simulink model "sampleModel7288_pp_1_1"  (R2018a)
settings: Solver=VariableStepAuto  StartTime=0.0  StopTime=10.0  RelTol=1e-3
undefined symbols (not defined in the file): DiscIntNeverNeededParam, sigbuilder_block
libraries: simulink x497
(part 4 of 10)

== system sampleModel7288_pp_1_1/cfblk286 ==
  cfblk1 : Inport
  Action Port : ActionPort  ActionType=then
  cfblk{10..13} (4 alike) : Delay
  cfblk3 : simulink/Continuous/PID Controller (2DOF)  Controller=PID  TimeDomain=Discrete-time  SampleTime=-1  IntegratorMethod=Forward Euler  FilterMethod=Forward Euler  Form=Parallel  UseFilter=on  ControllerParametersSource=internal  P=1  I=1  D=0  N=100  b=1  c=1  InitialConditionSource=internal  InitialConditionForIntegrator=0  InitialConditionForFilter=0  ExternalReset=none  LimitOutput=off  UpperSaturationLimit=inf  LowerSaturationLimit=-inf  LinearizeAsGain=off  AntiWindupMode=none  Kb=1  TrackingMode=off  Kt=1  PParamMin=[]  PParamMax=[]  IParamMin=[]  IParamMax=[]  DParamMin=[]  DParamMax=[]  NParamMin=[]  NParamMax=[]  bParamMin=[]  bParamMax=[]  cParamMin=[]  cParamMax=[]  KbParamMin=[]  KbParamMax=[]  KtParamMin=[]  KtParamMax=[]  POutMin=[]  POutMax=[]  IOutMin=[]  IOutMax=[]  DOutMin=[]  DOutMax=[]  NOutMin=[]  NOutMax=[]  bOutMin=[]  bOutMax=[]  cOutMin=[]  cOutMax=[]  KbOutMin=[]  KbOutMax=[]  KtOutMin=[]  KtOutMax=[]  IntegratorOutMin=[]  IntegratorOutMax=[]  FilterOutMin=[]  FilterOutMax=[]  SumOutMin=[]  SumOutMax=[]  Sum1OutMin=[]  Sum1OutMax=[]  Sum2OutMin=[]  Sum2OutMax=[]  Sum3OutMin=[]  Sum3OutMax=[]  SumI1OutMin=[]  SumI1OutMax=[]  SumI2OutMin=[]  SumI2OutMax=[]  SumI3OutMin=[]  SumI3OutMax=[]  SumDOutMin=[]  SumDOutMax=[]  SaturationOutMin=[]  SaturationOutMax=[]  IntegratorContinuousStateAttributes=''  IntegratorStateMustResolveToSignalObject=off  IntegratorRTWStateStorageClass=Auto  FilterContinuousStateAttributes=''  FilterStateMustResolveToSignalObject=off  FilterRTWStateStorageClass=Auto  DifferentiatorICPrevScaledInput=0  DifferentiatorOutMin=[]  DifferentiatorOutMax=[]  FilterDiffOutCoefMin=[]  FilterDiffOutCoefMax=[]  SumDenOutMin=[]  SumDenOutMax=[]  SumNumOutMin=[]  SumNumOutMax=[]  ReciprocalOutMin=[]  ReciprocalOutMax=[]  DivideOutMin=[]  DivideOutMax=[]  TunerSelectOption=Transfer Function Based (PID Tuner App)
  cfblk4 : DiscreteFilter
  cfblk5 : DiscreteZeroPole  Poles=[0 0.5]  Gain=1  SampleTime=-1
  cfblk6 : Delay  DelayLengthSource=Input port
      settings: InputPortMap=u0,p1
  cfblk7 : simulink/Continuous/PID Controller (2DOF)  Controller=PID  TimeDomain=Discrete-time  SampleTime=-1  IntegratorMethod=Forward Euler  FilterMethod=Forward Euler  Form=Parallel  UseFilter=on  ControllerParametersSource=internal  P=1  I=1  D=0  N=100  b=1  c=1  InitialConditionSource=internal  InitialConditionForIntegrator=0  InitialConditionForFilter=0  ExternalReset=none  LimitOutput=off  UpperSaturationLimit=inf  LowerSaturationLimit=-inf  LinearizeAsGain=off  AntiWindupMode=none  Kb=1  TrackingMode=off  Kt=1  PParamMin=[]  PParamMax=[]  IParamMin=[]  IParamMax=[]  DParamMin=[]  DParamMax=[]  NParamMin=[]  NParamMax=[]  bParamMin=[]  bParamMax=[]  cParamMin=[]  cParamMax=[]  KbParamMin=[]  KbParamMax=[]  KtParamMin=[]  KtParamMax=[]  POutMin=[]  POutMax=[]  IOutMin=[]  IOutMax=[]  DOutMin=[]  DOutMax=[]  NOutMin=[]  NOutMax=[]  bOutMin=[]  bOutMax=[]  cOutMin=[]  cOutMax=[]  KbOutMin=[]  KbOutMax=[]  KtOutMin=[]  KtOutMax=[]  IntegratorOutMin=[]  IntegratorOutMax=[]  FilterOutMin=[]  FilterOutMax=[]  SumOutMin=[]  SumOutMax=[]  Sum1OutMin=[]  Sum1OutMax=[]  Sum2OutMin=[]  Sum2OutMax=[]  Sum3OutMin=[]  Sum3OutMax=[]  SumI1OutMin=[]  SumI1OutMax=[]  SumI2OutMin=[]  SumI2OutMax=[]  SumI3OutMin=[]  SumI3OutMax=[]  SumDOutMin=[]  SumDOutMax=[]  SaturationOutMin=[]  SaturationOutMax=[]  IntegratorContinuousStateAttributes=''  IntegratorStateMustResolveToSignalObject=off  IntegratorRTWStateStorageClass=Auto  FilterContinuousStateAttributes=''  FilterStateMustResolveToSignalObject=off  FilterRTWStateStorageClass=Auto  DifferentiatorICPrevScaledInput=0  DifferentiatorOutMin=[]  DifferentiatorOutMax=[]  FilterDiffOutCoefMin=[]  FilterDiffOutCoefMax=[]  SumDenOutMin=[]  SumDenOutMax=[]  SumNumOutMin=[]  SumNumOutMax=[]  ReciprocalOutMin=[]  ReciprocalOutMax=[]  DivideOutMin=[]  DivideOutMax=[]  TunerSelectOption=Transfer Function Based (PID Tuner App)
  cyemi_{778..789} (12 alike) : DataTypeConversion  OutDataTypeStr=double
  cfblk2 : Outport
  cfblk8 : Outport  Port=2
  cfblk9 : Outport  Port=3
  wires:
  cfblk5/1 -> cfblk2/1, cyemi_778/1, cyemi_779/1, cyemi_784/1
  cfblk1/1 -> cfblk9/1
  cfblk6/1 -> cfblk8/1, cyemi_781/1, cyemi_785/1
  cyemi_778/1 -> cfblk10/1
  cyemi_779/1 -> cfblk11/1
  cyemi_780/1 -> cfblk12/1
  cfblk4/1 -> cyemi_780/1
  cyemi_781/1 -> cfblk13/1
  cyemi_782/1 -> cfblk3/1
  cfblk10/1 -> cyemi_782/1
  cyemi_783/1 -> cfblk3/2
  cfblk13/1 -> cyemi_783/1
  cyemi_784/1 -> cfblk4/1
  cyemi_785/1 -> cfblk5/1
  cyemi_786/1 -> cfblk6/1
  cfblk12/1 -> cyemi_786/1
  cyemi_787/1 -> cfblk6/2
  cfblk7/1 -> cyemi_787/1
  cyemi_788/1 -> cfblk7/1
  cfblk3/1 -> cyemi_788/1
  cyemi_789/1 -> cfblk7/2
  cfblk11/1 -> cyemi_789/1

== system sampleModel7288_pp_1_1/cfblk287 ==
  cfblk1 : Inport
  cfblk11 : Inport  Port=2
  cfblk12 : Inport  Port=3
  Action Port : ActionPort  ActionType=else
  cfblk10 : simulink/Continuous/PID Controller  Controller=PID  TimeDomain=Discrete-time  SampleTime=-1  IntegratorMethod=Forward Euler  FilterMethod=Forward Euler  Form=Parallel  UseFilter=on  ControllerParametersSource=internal  P=1  I=1  D=0  N=100  InitialConditionSource=internal  InitialConditionForIntegrator=0  InitialConditionForFilter=0  ExternalReset=none  LimitOutput=off  UpperSaturationLimit=inf  LowerSaturationLimit=-inf  LinearizeAsGain=off  AntiWindupMode=none  Kb=1  TrackingMode=off  Kt=1  PParamMin=[]  PParamMax=[]  IParamMin=[]  IParamMax=[]  DParamMin=[]  DParamMax=[]  NParamMin=[]  NParamMax=[]  KbParamMin=[]  KbParamMax=[]  KtParamMin=[]  KtParamMax=[]  POutMin=[]  POutMax=[]  IOutMin=[]  IOutMax=[]  DOutMin=[]  DOutMax=[]  NOutMin=[]  NOutMax=[]  KbOutMin=[]  KbOutMax=[]  KtOutMin=[]  KtOutMax=[]  IntegratorOutMin=[]  IntegratorOutMax=[]  FilterOutMin=[]  FilterOutMax=[]  SumOutMin=[]  SumOutMax=[]  SumI1OutMin=[]  SumI1OutMax=[]  SumI2OutMin=[]  SumI2OutMax=[]  SumI3OutMin=[]  SumI3OutMax=[]  SumDOutMin=[]  SumDOutMax=[]  SaturationOutMin=[]  SaturationOutMax=[]  IntegratorContinuousStateAttributes=''  IntegratorStateMustResolveToSignalObject=off  IntegratorRTWStateStorageClass=Auto  FilterContinuousStateAttributes=''  FilterStateMustResolveToSignalObject=off  FilterRTWStateStorageClass=Auto  DifferentiatorICPrevScaledInput=0  DifferentiatorOutMin=[]  DifferentiatorOutMax=[]  FilterDiffOutCoefMin=[]  FilterDiffOutCoefMax=[]  SumDenOutMin=[]  SumDenOutMax=[]  SumNumOutMin=[]  SumNumOutMax=[]  ReciprocalOutMin=[]  ReciprocalOutMax=[]  DivideOutMin=[]  DivideOutMax=[]  TunerSelectOption=Transfer Function Based (PID Tuner App)
  cfblk15 : Delay
  cfblk16 : Delay
  cfblk3 : DiscreteTransferFcn
  cfblk4 : DiscreteIntegrator  SampleTime=-1  OutDataTypeStr=double  ICPrevOutput=DiscIntNeverNeededParam  ICPrevScaledInput=DiscIntNeverNeededParam
  cfblk5 : Delay  DelayLengthSource=Input port
      settings: InputPortMap=u0,p1
  cfblk6 : Delay  DelayLengthSource=Input port
      settings: InputPortMap=u0,p1
  cfblk7 : simulink/Discrete/Tapped Delay  vinit=0.0  samptime=-1  NumDelays=1  DelayOrder=Oldest  includeCurrent=off
  cfblk8 : simulink/Discrete/Difference  ICPrevInput=0.0  OutMin=[]  OutMax=[]  OutDataTypeStr=double  OutputDataTypeScalingMode=double  OutDataType=fixdt(1, 16)  OutScaling=2^-10  DoSatur=off
  cfblk9 : DiscreteStateSpace  SampleTime=-1
  cyemi_{793..804} (12 alike) : DataTypeConversion  OutDataTypeStr=double
  cfblk2 : Outport
  cfblk13 : Outport  Port=2
  cfblk14 : Outport  Port=3
  wires:
  cfblk7/1 -> cfblk13/1
  cfblk11/1 -> cyemi_798/1, cyemi_802/1
  cfblk1/1 -> cfblk2/1
  cfblk9/1 -> cfblk14/1
  cfblk8/1 -> cyemi_795/1, cyemi_797/1
  cyemi_793/1 -> cfblk10/1
  cfblk5/1 -> cyemi_793/1
  cyemi_794/1 -> cfblk15/1
  cfblk6/1 -> cyemi_794/1
  cyemi_795/1 -> cfblk16/1
  cyemi_796/1 -> cfblk3/1
  cfblk15/1 -> cyemi_796/1
  cyemi_797/1 -> cfblk4/1
  cyemi_798/1 -> cfblk5/1
  cyemi_799/1 -> cfblk5/2
  cfblk16/1 -> cyemi_799/1
  cyemi_800/1 -> cfblk6/1
  cfblk3/1 -> cyemi_800/1
  cyemi_801/1 -> cfblk6/2
  cfblk12/1 -> cyemi_801/1
  cyemi_802/1 -> cfblk7/1
  cyemi_803/1 -> cfblk8/1
  cfblk10/1 -> cyemi_803/1
  cyemi_804/1 -> cfblk9/1
  cfblk4/1 -> cyemi_804/1

== system sampleModel7288_pp_1_1/cfblk288 ==
  cfblk1 : Inport
  cfblk11 : Inport  Port=2
  Action Port : ActionPort  ActionType=then
  cfblk10 : If  SampleTime=1
  cfblk15 : Subsystem  TreatAsAtomicUnit=on
  cfblk16 : Subsystem  TreatAsAtomicUnit=on
  cfblk17 : Delay
  cfblk18 : Delay
  cfblk19 : Delay
  cfblk3 : simulink/Continuous/PID Controller  Controller=PID  TimeDomain=Discrete-time  SampleTime=-1  IntegratorMethod=Forward Euler  FilterMethod=Forward Euler  Form=Parallel  UseFilter=on  ControllerParametersSource=internal  P=1  I=1  D=0  N=100  InitialConditionSource=internal  InitialConditionForIntegrator=0  InitialConditionForFilter=0  ExternalReset=none  LimitOutput=off  UpperSaturationLimit=inf  LowerSaturationLimit=-inf  LinearizeAsGain=off  AntiWindupMode=none  Kb=1  TrackingMode=off  Kt=1  PParamMin=[]  PParamMax=[]  IParamMin=[]  IParamMax=[]  DParamMin=[]  DParamMax=[]  NParamMin=[]  NParamMax=[]  KbParamMin=[]  KbParamMax=[]  KtParamMin=[]  KtParamMax=[]  POutMin=[]  POutMax=[]  IOutMin=[]  IOutMax=[]  DOutMin=[]  DOutMax=[]  NOutMin=[]  NOutMax=[]  KbOutMin=[]  KbOutMax=[]  KtOutMin=[]  KtOutMax=[]  IntegratorOutMin=[]  IntegratorOutMax=[]  FilterOutMin=[]  FilterOutMax=[]  SumOutMin=[]  SumOutMax=[]  SumI1OutMin=[]  SumI1OutMax=[]  SumI2OutMin=[]  SumI2OutMax=[]  SumI3OutMin=[]  SumI3OutMax=[]  SumDOutMin=[]  SumDOutMax=[]  SaturationOutMin=[]  SaturationOutMax=[]  IntegratorContinuousStateAttributes=''  IntegratorStateMustResolveToSignalObject=off  IntegratorRTWStateStorageClass=Auto  FilterContinuousStateAttributes=''  FilterStateMustResolveToSignalObject=off  FilterRTWStateStorageClass=Auto  DifferentiatorICPrevScaledInput=0  DifferentiatorOutMin=[]  DifferentiatorOutMax=[]  FilterDiffOutCoefMin=[]  FilterDiffOutCoefMax=[]  SumDenOutMin=[]  SumDenOutMax=[]  SumNumOutMin=[]  SumNumOutMax=[]  ReciprocalOutMin=[]  ReciprocalOutMax=[]  DivideOutMin=[]  DivideOutMax=[]  TunerSelectOption=Transfer Function Based (PID Tuner App)
  cfblk4 : DiscreteStateSpace  SampleTime=-1
  cfblk5 : simulink/Discrete/Tapped Delay  vinit=0.0  samptime=-1  NumDelays=1  DelayOrder=Oldest  includeCurrent=off
  cfblk6 : Delay  DelayLengthSource=Input port
      settings: InputPortMap=u0,p1
  cfblk7 : Delay  DelayLengthSource=Input port
      settings: InputPortMap=u0,p1
  cfblk8 : UnitDelay  SampleTime=-1
  cfblk9 : UnitDelay  SampleTime=-1
  cyemi_{807..808,820..821,828..834,836..839} (15 alike) : DataTypeConversion  OutDataTypeStr=double
  cyemi_835 : DataTypeConversion  OutDataTypeStr=uint32
  cfblk2 : Outport
  cfblk12 : Outport  Port=2
  cfblk13 : Outport  Port=3
  cfblk14 : Outport  Port=4
  wires:
  cfblk15/1(cfblk2) -> cfblk2/1
  cfblk6/1 -> cyemi_828/1, cyemi_839/1
  cfblk9/1 -> cfblk12/1, cyemi_838/1
  cfblk8/1 -> cfblk13/1
  cfblk15/2(cfblk11) -> cyemi_829/1, cyemi_837/1
  cfblk3/1 -> cfblk14/1, cyemi_821/1, cyemi_836/1
  cfblk10/1 -> cfblk15/Action
  cfblk10/2 -> cfblk16/Action
  cyemi_807/1 -> cfblk10/1
  cfblk19/1 -> cyemi_807/1
  cyemi_808/1 -> cfblk15/1(cfblk1)
  cfblk17/1 -> cyemi_808/1
  cyemi_820/1 -> cfblk16/1(cfblk1)
  cfblk18/1 -> cyemi_820/1
  cyemi_821/1 -> cfblk16/2(cfblk8)
  cyemi_828/1 -> cfblk17/1
  cyemi_829/1 -> cfblk18/1
  cyemi_830/1 -> cfblk19/1
  cfblk4/1 -> cyemi_830/1
  cyemi_831/1 -> cfblk3/1
  cfblk5/1 -> cyemi_831/1
  cyemi_832/1 -> cfblk4/1
  cfblk7/1 -> cyemi_832/1
  cyemi_833/1 -> cfblk5/1
  cfblk1/1 -> cyemi_833/1
  cyemi_834/1 -> cfblk6/1
  cfblk16/1(cfblk2) -> cyemi_834/1
  cyemi_835/1 -> cfblk6/2
  cfblk11/1 -> cyemi_835/1
  cyemi_836/1 -> cfblk7/1
  cyemi_837/1 -> cfblk7/2
  cyemi_838/1 -> cfblk8/1
  cyemi_839/1 -> cfblk9/1

== system sampleModel7288_pp_1_1/cfblk289 ==
  cfblk1 : Inport
  Action Port : ActionPort  ActionType=else
  cfblk3 : simulink/Continuous/PID Controller  Controller=PID  TimeDomain=Discrete-time  SampleTime=-1  IntegratorMethod=Forward Euler  FilterMethod=Forward Euler  Form=Parallel  UseFilter=on  ControllerParametersSource=internal  P=1  I=1  D=0  N=100  InitialConditionSource=internal  InitialConditionForIntegrator=0  InitialConditionForFilter=0  ExternalReset=none  LimitOutput=off  UpperSaturationLimit=inf  LowerSaturationLimit=-inf  LinearizeAsGain=off  AntiWindupMode=none  Kb=1  TrackingMode=off  Kt=1  PParamMin=[]  PParamMax=[]  IParamMin=[]  IParamMax=[]  DParamMin=[]  DParamMax=[]  NParamMin=[]  NParamMax=[]  KbParamMin=[]  KbParamMax=[]  KtParamMin=[]  KtParamMax=[]  POutMin=[]  POutMax=[]  IOutMin=[]  IOutMax=[]  DOutMin=[]  DOutMax=[]  NOutMin=[]  NOutMax=[]  KbOutMin=[]  KbOutMax=[]  KtOutMin=[]  KtOutMax=[]  IntegratorOutMin=[]  IntegratorOutMax=[]  FilterOutMin=[]  FilterOutMax=[]  SumOutMin=[]  SumOutMax=[]  SumI1OutMin=[]  SumI1OutMax=[]  SumI2OutMin=[]  SumI2OutMax=[]  SumI3OutMin=[]  SumI3OutMax=[]  SumDOutMin=[]  SumDOutMax=[]  SaturationOutMin=[]  SaturationOutMax=[]  IntegratorContinuousStateAttributes=''  IntegratorStateMustResolveToSignalObject=off  IntegratorRTWStateStorageClass=Auto  FilterContinuousStateAttributes=''  FilterStateMustResolveToSignalObject=off  FilterRTWStateStorageClass=Auto  DifferentiatorICPrevScaledInput=0  DifferentiatorOutMin=[]  DifferentiatorOutMax=[]  FilterDiffOutCoefMin=[]  FilterDiffOutCoefMax=[]  SumDenOutMin=[]  SumDenOutMax=[]  SumNumOutMin=[]  SumNumOutMax=[]  ReciprocalOutMin=[]  ReciprocalOutMax=[]  DivideOutMin=[]  DivideOutMax=[]  TunerSelectOption=Transfer Function Based (PID Tuner App)
  cfblk4 : DiscreteStateSpace  SampleTime=-1
  cfblk5 : DiscreteStateSpace  SampleTime=-1
  cfblk6 : simulink/Discrete/Tapped Delay  vinit=0.0  samptime=-1  NumDelays=1  DelayOrder=Oldest  includeCurrent=off
  cfblk7 : DiscreteIntegrator  SampleTime=-1  OutDataTypeStr=double  ICPrevOutput=DiscIntNeverNeededParam  ICPrevScaledInput=DiscIntNeverNeededParam
  cfblk8 : Delay  ShowEnablePort=on
      settings: InputPortMap=u0,e6
  cyemi_{841..847} (7 alike) : DataTypeConversion  OutDataTypeStr=double
  cfblk2 : Outport
  cfblk9 : Outport  Port=2
  wires:
  cfblk3/1 -> cyemi_845/1, cyemi_846/1
  cfblk4/1 -> cyemi_841/1, cyemi_847/1
  cfblk7/1 -> cfblk9/1
  cfblk8/1 -> cfblk2/1
  cyemi_841/1 -> cfblk3/1
  cyemi_842/1 -> cfblk4/1
  cfblk5/1 -> cyemi_842/1
  cyemi_843/1 -> cfblk5/1
  cfblk6/1 -> cyemi_843/1
  cyemi_844/1 -> cfblk6/1
  cfblk1/1 -> cyemi_844/1
  cyemi_845/1 -> cfblk7/1
  cyemi_846/1 -> cfblk8/1
  cyemi_847/1 -> cfblk8/2

== system sampleModel7288_pp_1_1/cfblk290 ==
  cfblk1 : Inport
  cfblk12 : Inport  Port=2
  Action Port : ActionPort  ActionType=then
  cfblk10 : Delay  ShowEnablePort=on
      settings: InputPortMap=u0,e6
  cfblk11 : DiscreteFir
  cfblk14 : Delay
  cfblk3 : DiscreteFilter
  cfblk4 : DiscreteFir
  cfblk5 : simulink/Discrete/Transfer Fcn Real Zero  ZeroZ=0.75  ICPrevInput=0.0  DoSatur=off
      settings: SourceProductName=Simulink  SourceProductBaseCode=SL
  cfblk6 : UnitDelay  SampleTime=-1
  cfblk7 : simulink/Discrete/Transfer Fcn First Order  PoleZ=0.95  ICPrevOutput=0.0  DoSatur=off
      settings: SourceProductName=Simulink
  cfblk8 : simulink/Continuous/PID Controller  Controller=PID  TimeDomain=Discrete-time  SampleTime=-1  IntegratorMethod=Forward Euler  FilterMethod=Forward Euler  Form=Parallel  UseFilter=on  ControllerParametersSource=internal  P=1  I=1  D=0  N=100  InitialConditionSource=internal  InitialConditionForIntegrator=0  InitialConditionForFilter=0  ExternalReset=none  LimitOutput=off  UpperSaturationLimit=inf  LowerSaturationLimit=-inf  LinearizeAsGain=off  AntiWindupMode=none  Kb=1  TrackingMode=off  Kt=1  PParamMin=[]  PParamMax=[]  IParamMin=[]  IParamMax=[]  DParamMin=[]  DParamMax=[]  NParamMin=[]  NParamMax=[]  KbParamMin=[]  KbParamMax=[]  KtParamMin=[]  KtParamMax=[]  POutMin=[]  POutMax=[]  IOutMin=[]  IOutMax=[]  DOutMin=[]  DOutMax=[]  NOutMin=[]  NOutMax=[]  KbOutMin=[]  KbOutMax=[]  KtOutMin=[]  KtOutMax=[]  IntegratorOutMin=[]  IntegratorOutMax=[]  FilterOutMin=[]  FilterOutMax=[]  SumOutMin=[]  SumOutMax=[]  SumI1OutMin=[]  SumI1OutMax=[]  SumI2OutMin=[]  SumI2OutMax=[]  SumI3OutMin=[]  SumI3OutMax=[]  SumDOutMin=[]  SumDOutMax=[]  SaturationOutMin=[]  SaturationOutMax=[]  IntegratorContinuousStateAttributes=''  IntegratorStateMustResolveToSignalObject=off  IntegratorRTWStateStorageClass=Auto  FilterContinuousStateAttributes=''  FilterStateMustResolveToSignalObject=off  FilterRTWStateStorageClass=Auto  DifferentiatorICPrevScaledInput=0  DifferentiatorOutMin=[]  DifferentiatorOutMax=[]  FilterDiffOutCoefMin=[]  FilterDiffOutCoefMax=[]  SumDenOutMin=[]  SumDenOutMax=[]  SumNumOutMin=[]  SumNumOutMax=[]  ReciprocalOutMin=[]  ReciprocalOutMax=[]  DivideOutMin=[]  DivideOutMax=[]  TunerSelectOption=Transfer Function Based (PID Tuner App)
  cfblk9 : simulink/Discrete/Transfer Fcn Lead or Lag  PoleZ=0.95  ZeroZ=0.75  ICPrevOutput=0.0  ICPrevInput=0.0  DoSatur=off
      settings: SourceProductName=Simulink  SourceProductBaseCode=SL
  cyemi_{851..861} (11 alike) : DataTypeConversion  OutDataTypeStr=double
  cfblk2 : Outport
  cfblk13 : Outport  Port=2
  wires:
  cfblk10/1 -> cfblk2/1
  cfblk7/1 -> cfblk13/1
  cfblk1/1 -> cyemi_852/1, cyemi_856/1
  cyemi_851/1 -> cfblk10/1
  cfblk11/1 -> cyemi_851/1
  cyemi_852/1 -> cfblk10/2
  cyemi_853/1 -> cfblk11/1
  cfblk8/1 -> cyemi_853/1
  cyemi_854/1 -> cfblk14/1
  cfblk9/1 -> cyemi_854/1
  cyemi_855/1 -> cfblk3/1
  cfblk12/1 -> cyemi_855/1
  cyemi_856/1 -> cfblk4/1
  cyemi_857/1 -> cfblk5/1
  cfblk4/1 -> cyemi_857/1
  cyemi_858/1 -> cfblk6/1
  cfblk14/1 -> cyemi_858/1
  cyemi_859/1 -> cfblk7/1
  cfblk3/1 -> cyemi_859/1
  cyemi_860/1 -> cfblk8/1
  cfblk5/1 -> cyemi_860/1
  cyemi_861/1 -> cfblk9/1
  cfblk6/1 -> cyemi_861/1

== system sampleModel7288_pp_1_1/cfblk291 ==
  cfblk1 : Inport
  cfblk11 : Inport  Port=2
  Action Port : ActionPort  ActionType=else
  cfblk10 : DiscreteStateSpace  SampleTime=-1
  cfblk14 : Delay
  cfblk15 : DataTypeConversion  OutDataTypeStr=uint32
  cfblk16 : DataTypeConversion  OutDataTypeStr=double
  cfblk17 : DataTypeConversion  OutDataTypeStr=double
  cfblk18 : DataTypeConversion  OutDataTypeStr=uint32
  cfblk3 : simulink/Continuous/PID Controller  Controller=PID  TimeDomain=Discrete-time  SampleTime=-1  IntegratorMethod=Forward Euler  FilterMethod=Forward Euler  Form=Parallel  UseFilter=on  ControllerParametersSource=internal  P=1  I=1  D=0  N=100  InitialConditionSource=internal  InitialConditionForIntegrator=0  InitialConditionForFilter=0  ExternalReset=none  LimitOutput=off  UpperSaturationLimit=inf  LowerSaturationLimit=-inf  LinearizeAsGain=off  AntiWindupMode=none  Kb=1  TrackingMode=off  Kt=1  PParamMin=[]  PParamMax=[]  IParamMin=[]  IParamMax=[]  DParamMin=[]  DParamMax=[]  NParamMin=[]  NParamMax=[]  KbParamMin=[]  KbParamMax=[]  KtParamMin=[]  KtParamMax=[]  POutMin=[]  POutMax=[]  IOutMin=[]  IOutMax=[]  DOutMin=[]  DOutMax=[]  NOutMin=[]  NOutMax=[]  KbOutMin=[]  KbOutMax=[]  KtOutMin=[]  KtOutMax=[]  IntegratorOutMin=[]  IntegratorOutMax=[]  FilterOutMin=[]  FilterOutMax=[]  SumOutMin=[]  SumOutMax=[]  SumI1OutMin=[]  SumI1OutMax=[]  SumI2OutMin=[]  SumI2OutMax=[]  SumI3OutMin=[]  SumI3OutMax=[]  SumDOutMin=[]  SumDOutMax=[]  SaturationOutMin=[]  SaturationOutMax=[]  IntegratorContinuousStateAttributes=''  IntegratorStateMustResolveToSignalObject=off  IntegratorRTWStateStorageClass=Auto  FilterContinuousStateAttributes=''  FilterStateMustResolveToSignalObject=off  FilterRTWStateStorageClass=Auto  DifferentiatorICPrevScaledInput=0  DifferentiatorOutMin=[]  DifferentiatorOutMax=[]  FilterDiffOutCoefMin=[]  FilterDiffOutCoefMax=[]  SumDenOutMin=[]  SumDenOutMax=[]  SumNumOutMin=[]  SumNumOutMax=[]  ReciprocalOutMin=[]  ReciprocalOutMax=[]  DivideOutMin=[]  DivideOutMax=[]  TunerSelectOption=Transfer Function Based (PID Tuner App)
  cfblk4 : Delay  DelayLengthSource=Input port
      settings: InputPortMap=u0,p1
  cfblk5 : simulink/Discrete/Tapped Delay  vinit=0.0  samptime=-1  NumDelays=1  DelayOrder=Oldest  includeCurrent=off
  cfblk6 : Delay  DelayLengthSource=Input port
      settings: InputPortMap=u0,p1
  cfblk7 : DiscreteFilter
  cfblk8 : simulink/Discrete/Transfer Fcn First Order  PoleZ=0.95  ICPrevOutput=0.0  DoSatur=off
      settings: SourceProductName=Simulink
  cfblk9 : DiscreteZeroPole  Poles=[0 0.5]  Gain=1  SampleTime=-1
  cyemi_{864..871,873..878} (14 alike) : DataTypeConversion  OutDataTypeStr=double
  cyemi_872 : DataTypeConversion  OutDataTypeStr=uint32
  cfblk2 : Outport
  cfblk12 : Outport  Port=2
  cfblk13 : Outport  Port=3
  wires:
  cfblk3/1 -> cfblk2/1
  cfblk9/1 -> cyemi_865/1, cyemi_866/1
  cfblk6/1 -> cfblk13/1
  cfblk8/1 -> cyemi_864/1, cyemi_873/1
  cfblk10/1 -> cyemi_869/1, cyemi_878/1
  cfblk15/1 -> cfblk12/1
  cyemi_864/1 -> cfblk10/1
  cyemi_865/1 -> cfblk14/1
  cyemi_866/1 -> cfblk15/1
  cyemi_867/1 -> cfblk16/1
  cfblk4/1 -> cyemi_867/1
  cyemi_868/1 -> cfblk17/1
  cfblk1/1 -> cyemi_868/1
  cyemi_869/1 -> cfblk18/1
  cyemi_870/1 -> cfblk3/1
  cfblk11/1 -> cyemi_870/1
  cyemi_871/1 -> cfblk4/1
  cfblk17/1 -> cyemi_871/1
  cyemi_872/1 -> cfblk4/2
  cfblk18/1 -> cyemi_872/1
  cyemi_873/1 -> cfblk5/1
  cyemi_874/1 -> cfblk6/1
  cfblk16/1 -> cyemi_874/1
  cyemi_875/1 -> cfblk6/2
  cfblk7/1 -> cyemi_875/1
  cyemi_876/1 -> cfblk7/1
  cfblk5/1 -> cyemi_876/1
  cyemi_877/1 -> cfblk8/1
  cfblk14/1 -> cyemi_877/1
  cyemi_878/1 -> cfblk9/1

== system sampleModel7288_pp_1_1/cfblk292 ==
  cfblk1 : Inport
  Action Port : ActionPort  ActionType=then
  cfblk10 : DiscreteFir
  cfblk11 : simulink/Discrete/Transfer Fcn First Order  PoleZ=0.95  ICPrevOutput=0.0  DoSatur=off
      settings: SourceProductName=Simulink
  cfblk14 : Delay
  cfblk3 : simulink/Continuous/PID Controller  Controller=PID  TimeDomain=Discrete-time  SampleTime=-1  IntegratorMethod=Forward Euler  FilterMethod=Forward Euler  Form=Parallel  UseFilter=on  ControllerParametersSource=internal  P=1  I=1  D=0  N=100  InitialConditionSource=internal  InitialConditionForIntegrator=0  InitialConditionForFilter=0  ExternalReset=none  LimitOutput=off  UpperSaturationLimit=inf  LowerSaturationLimit=-inf  LinearizeAsGain=off  AntiWindupMode=none  Kb=1  TrackingMode=off  Kt=1  PParamMin=[]  PParamMax=[]  IParamMin=[]  IParamMax=[]  DParamMin=[]  DParamMax=[]  NParamMin=[]  NParamMax=[]  KbParamMin=[]  KbParamMax=[]  KtParamMin=[]  KtParamMax=[]  POutMin=[]  POutMax=[]  IOutMin=[]  IOutMax=[]  DOutMin=[]  DOutMax=[]  NOutMin=[]  NOutMax=[]  KbOutMin=[]  KbOutMax=[]  KtOutMin=[]  KtOutMax=[]  IntegratorOutMin=[]  IntegratorOutMax=[]  FilterOutMin=[]  FilterOutMax=[]  SumOutMin=[]  SumOutMax=[]  SumI1OutMin=[]  SumI1OutMax=[]  SumI2OutMin=[]  SumI2OutMax=[]  SumI3OutMin=[]  SumI3OutMax=[]  SumDOutMin=[]  SumDOutMax=[]  SaturationOutMin=[]  SaturationOutMax=[]  IntegratorContinuousStateAttributes=''  IntegratorStateMustResolveToSignalObject=off  IntegratorRTWStateStorageClass=Auto  FilterContinuousStateAttributes=''  FilterStateMustResolveToSignalObject=off  FilterRTWStateStorageClass=Auto  DifferentiatorICPrevScaledInput=0  DifferentiatorOutMin=[]  DifferentiatorOutMax=[]  FilterDiffOutCoefMin=[]  FilterDiffOutCoefMax=[]  SumDenOutMin=[]  SumDenOutMax=[]  SumNumOutMin=[]  SumNumOutMax=[]  ReciprocalOutMin=[]  ReciprocalOutMax=[]  DivideOutMin=[]  DivideOutMax=[]  TunerSelectOption=Transfer Function Based (PID Tuner App)
  cfblk4 : DiscreteZeroPole  Poles=[0 0.5]  Gain=1  SampleTime=-1
  cfblk5 : Delay  ShowEnablePort=on
      settings: InputPortMap=u0,e6
  cfblk6 : simulink/Continuous/PID Controller  Controller=PID  TimeDomain=Discrete-time  SampleTime=-1  IntegratorMethod=Forward Euler  FilterMethod=Forward Euler  Form=Parallel  UseFilter=on  ControllerParametersSource=internal  P=1  I=1  D=0  N=100  InitialConditionSource=internal  InitialConditionForIntegrator=0  InitialConditionForFilter=0  ExternalReset=none  LimitOutput=off  UpperSaturationLimit=inf  LowerSaturationLimit=-inf  LinearizeAsGain=off  AntiWindupMode=none  Kb=1  TrackingMode=off  Kt=1  PParamMin=[]  PParamMax=[]  IParamMin=[]  IParamMax=[]  DParamMin=[]  DParamMax=[]  NParamMin=[]  NParamMax=[]  KbParamMin=[]  KbParamMax=[]  KtParamMin=[]  KtParamMax=[]  POutMin=[]  POutMax=[]  IOutMin=[]  IOutMax=[]  DOutMin=[]  DOutMax=[]  NOutMin=[]  NOutMax=[]  KbOutMin=[]  KbOutMax=[]  KtOutMin=[]  KtOutMax=[]  IntegratorOutMin=[]  IntegratorOutMax=[]  FilterOutMin=[]  FilterOutMax=[]  SumOutMin=[]  SumOutMax=[]  SumI1OutMin=[]  SumI1OutMax=[]  SumI2OutMin=[]  SumI2OutMax=[]  SumI3OutMin=[]  SumI3OutMax=[]  SumDOutMin=[]  SumDOutMax=[]  SaturationOutMin=[]  SaturationOutMax=[]  IntegratorContinuousStateAttributes=''  IntegratorStateMustResolveToSignalObject=off  IntegratorRTWStateStorageClass=Auto  FilterContinuousStateAttributes=''  FilterStateMustResolveToSignalObject=off  FilterRTWStateStorageClass=Auto  DifferentiatorICPrevScaledInput=0  DifferentiatorOutMin=[]  DifferentiatorOutMax=[]  FilterDiffOutCoefMin=[]  FilterDiffOutCoefMax=[]  SumDenOutMin=[]  SumDenOutMax=[]  SumNumOutMin=[]  SumNumOutMax=[]  ReciprocalOutMin=[]  ReciprocalOutMax=[]  DivideOutMin=[]  DivideOutMax=[]  TunerSelectOption=Transfer Function Based (PID Tuner App)
  cfblk7 : DiscreteFilter
  cfblk8 : DiscreteTransferFcn
  cfblk9 : simulink/Discrete/Tapped Delay  vinit=0.0  samptime=-1  NumDelays=1  DelayOrder=Oldest  includeCurrent=off
  cyemi_{880..890} (11 alike) : DataTypeConversion  OutDataTypeStr=double
  cfblk2 : Outport
  cfblk12 : Outport  Port=2
  cfblk13 : Outport  Port=3
  wires:
  cfblk10/1 -> cyemi_882/1, cyemi_887/1
  cfblk5/1 -> cfblk2/1
  cfblk9/1 -> cfblk12/1, cyemi_886/1
  cfblk3/1 -> cfblk13/1
  cfblk1/1 -> cyemi_889/1, cyemi_890/1
  cyemi_880/1 -> cfblk10/1
  cfblk7/1 -> cyemi_880/1
  cyemi_881/1 -> cfblk11/1
  cfblk6/1 -> cyemi_881/1
  cyemi_882/1 -> cfblk14/1
  cyemi_883/1 -> cfblk3/1
  cfblk8/1 -> cyemi_883/1
  cyemi_884/1 -> cfblk4/1
  cfblk14/1 -> cyemi_884/1
  cyemi_885/1 -> cfblk5/1
  cfblk11/1 -> cyemi_885/1
  cyemi_886/1 -> cfblk5/2
  cyemi_887/1 -> cfblk6/1
  cyemi_888/1 -> cfblk7/1
  cfblk4/1 -> cyemi_888/1
  cyemi_889/1 -> cfblk8/1
  cyemi_890/1 -> cfblk9/1

== system sampleModel7288_pp_1_1/cfblk293 ==
  cfblk1 : Inport
  cfblk9 : Inport  Port=2
  cfblk10 : Inport  Port=3
  Action Port : ActionPort  ActionType=else
  cfblk11 : Subsystem  TreatAsAtomicUnit=on
  cfblk12 : Subsystem  TreatAsAtomicUnit=on
  cfblk13 : Delay
  cfblk14 : Delay
  cfblk15 : Delay
  cfblk3 : UnitDelay  SampleTime=-1
  cfblk4 : Delay  DelayLengthSource=Input port
      settings: InputPortMap=u0,p1
  cfblk5 : Delay  DelayLengthSource=Input port
      settings: InputPortMap=u0,p1
  cfblk6 : simulink/Discrete/Transfer Fcn Real Zero  ZeroZ=0.75  ICPrevInput=0.0  DoSatur=off
      settings: SourceProductName=Simulink  SourceProductBaseCode=SL
  cfblk7 : UnitDelay  SampleTime=-1
  cfblk8 : If  SampleTime=1
  cyemi_{894..896,910..911,917..927} (16 alike) : DataTypeConversion  OutDataTypeStr=double
  cfblk2 : Outport
  wires:
  cfblk1/1 -> cyemi_896/1, cyemi_926/1
  cfblk4/1 -> cfblk2/1
  cfblk8/1 -> cfblk11/Action
  cfblk8/2 -> cfblk12/Action
  cyemi_894/1 -> cfblk11/1(cfblk1)
  cfblk15/1 -> cyemi_894/1
  cyemi_895/1 -> cfblk11/2(cfblk14)
  cfblk9/1 -> cyemi_895/1
  cyemi_896/1 -> cfblk11/3(cfblk15)
  cyemi_910/1 -> cfblk12/1(cfblk1)
  cfblk7/1 -> cyemi_910/1
  cyemi_911/1 -> cfblk12/2(cfblk6)
  cfblk13/1 -> cyemi_911/1
  cyemi_917/1 -> cfblk13/1
  cfblk11/1(cfblk2) -> cyemi_917/1
  cyemi_918/1 -> cfblk14/1
  cfblk12/1(cfblk2) -> cyemi_918/1
  cyemi_919/1 -> cfblk15/1
  cfblk5/1 -> cyemi_919/1
  cyemi_920/1 -> cfblk3/1
  cfblk12/3(cfblk8) -> cyemi_920/1
  cyemi_921/1 -> cfblk4/1
  cfblk6/1 -> cyemi_921/1
  cyemi_922/1 -> cfblk4/2
  cfblk11/2(cfblk16) -> cyemi_922/1
  cyemi_923/1 -> cfblk5/1
  cfblk12/2(cfblk7) -> cyemi_923/1
  cyemi_924/1 -> cfblk5/2
  cfblk10/1 -> cyemi_924/1
  cyemi_925/1 -> cfblk6/1
  cfblk3/1 -> cyemi_925/1
  cyemi_926/1 -> cfblk7/1
  cyemi_927/1 -> cfblk8/1
  cfblk14/1 -> cyemi_927/1

== system sampleModel7288_pp_1_1/cfblk294 ==
  cfblk1 : Inport
  cfblk7 : Inport  Port=2
  cfblk8 : Inport  Port=3
  Action Port : ActionPort  ActionType=then
  cfblk3 : DiscreteFir
  cfblk4 : simulink/Discrete/Transfer Fcn Lead or Lag  PoleZ=0.95  ZeroZ=0.75  ICPrevOutput=0.0  ICPrevInput=0.0  DoSatur=off
      settings: SourceProductName=Simulink  SourceProductBaseCode=SL
  cfblk5 : simulink/Discrete/Tapped Delay  vinit=0.0  samptime=-1  NumDelays=1  DelayOrder=Oldest  includeCurrent=off
  cfblk6 : Delay
  cyemi_{931..934} (4 alike) : DataTypeConversion  OutDataTypeStr=double
  cfblk2 : Outport
  wires:
  cfblk7/1 -> cfblk2/1
  cyemi_931/1 -> cfblk3/1
  cfblk4/1 -> cyemi_931/1
  cyemi_932/1 -> cfblk4/1
  cfblk5/1 -> cyemi_932/1
  cyemi_933/1 -> cfblk5/1
  cfblk1/1 -> cyemi_933/1
  cyemi_934/1 -> cfblk6/1
  cfblk8/1 -> cyemi_934/1

== system sampleModel7288_pp_1_1/cfblk295 ==
  cfblk1 : Inport
  cfblk6 : Inport  Port=2
  cfblk7 : Inport  Port=3
  cfblk8 : Inport  Port=4
  Action Port : ActionPort  ActionType=else
  cfblk10 : Subsystem  TreatAsAtomicUnit=on
  cfblk11 : Subsystem  TreatAsAtomicUnit=on
  cfblk12 : Delay
  cfblk3 : UnitDelay  SampleTime=-1
  cfblk4 : simulink/Discrete/Difference  ICPrevInput=0.0  OutMin=[]  OutMax=[]  OutDataTypeStr=double  OutputDataTypeScalingMode=double  OutDataType=fixdt(1, 16)  OutScaling=2^-10  DoSatur=off
  cfblk5 : If  SampleTime=1
  cyemi_{939,953..955,963,965} (6 alike) : DataTypeConversion  OutDataTypeStr=double
  cyemi_964 : DataTypeConversion  OutDataTypeStr=uint8
  cyemi_966 : DataTypeConversion  OutDataTypeStr=uint8
  cfblk2 : Outport
  cfblk9 : Outport  Port=2
  wires:
  cfblk8/1 -> cfblk2/1
  cfblk4/1 -> cfblk9/1
  cfblk5/1 -> cfblk10/Action
  cfblk5/2 -> cfblk11/Action
  cyemi_939/1 -> cfblk10/1(cfblk1)
  cfblk12/1 -> cyemi_939/1
  cyemi_953/1 -> cfblk11/1(cfblk1)
  cfblk10/1(cfblk2) -> cyemi_953/1
  cyemi_954/1 -> cfblk11/2(cfblk8)
  cfblk10/2(cfblk13) -> cyemi_954/1
  cyemi_955/1 -> cfblk11/3(cfblk9)
  cfblk6/1 -> cyemi_955/1
  cyemi_963/1 -> cfblk12/1
  cfblk11/2(cfblk10) -> cyemi_963/1
  cyemi_964/1 -> cfblk3/1
  cfblk1/1 -> cyemi_964/1
  cyemi_965/1 -> cfblk4/1
  cfblk11/1(cfblk2) -> cyemi_965/1
  cyemi_966/1 -> cfblk5/1
  cfblk3/1 -> cyemi_966/1

== system sampleModel7288_pp_1_1/cfblk296 ==
  cfblk1 : Inport
  Action Port : ActionPort  ActionType=then
  cfblk10 : Subsystem  TreatAsAtomicUnit=on
  cfblk{11..14} (4 alike) : Delay
  cfblk3 : simulink/Discrete/Transfer Fcn First Order  PoleZ=0.95  ICPrevOutput=0.0  DoSatur=off
      settings: SourceProductName=Simulink
  cfblk4 : DiscreteZeroPole  Poles=[0 0.5]  Gain=1  SampleTime=-1
  cfblk5 : UnitDelay  SampleTime=-1
  cfblk6 : UnitDelay  SampleTime=-1
  cfblk7 : DiscreteZeroPole  Poles=[0 0.5]  Gain=1  SampleTime=-1
  cfblk8 : If  SampleTime=1
  cfblk9 : Subsystem  TreatAsAtomicUnit=on
  cyemi_{968..971,984..995} (16 alike) : DataTypeConversion  OutDataTypeStr=double
  cfblk2 : Outport
  wires:
  cfblk5/1 -> cfblk2/1, cyemi_985/1
  cfblk8/1 -> cfblk9/Action
  cfblk8/2 -> cfblk10/Action
  cyemi_968/1 -> cfblk10/1(cfblk1)
  cfblk11/1 -> cyemi_968/1
  cyemi_969/1 -> cfblk10/2(cfblk13)
  cfblk9/2(cfblk16) -> cyemi_969/1
  cyemi_970/1 -> cfblk10/3(cfblk14)
  cfblk9/3(cfblk17) -> cyemi_970/1
  cyemi_971/1 -> cfblk10/4(cfblk15)
  cfblk12/1 -> cyemi_971/1
  cyemi_984/1 -> cfblk11/1
  cfblk3/1 -> cyemi_984/1
  cyemi_985/1 -> cfblk12/1
  cyemi_986/1 -> cfblk13/1
  cfblk10/2(cfblk16) -> cyemi_986/1
  cyemi_987/1 -> cfblk14/1
  cfblk10/3(cfblk17) -> cyemi_987/1
  cyemi_988/1 -> cfblk3/1
  cfblk9/1(cfblk2) -> cyemi_988/1
  cyemi_989/1 -> cfblk4/1
  cfblk6/1 -> cyemi_989/1
  cyemi_990/1 -> cfblk5/1
  cfblk10/1(cfblk2) -> cyemi_990/1
  cyemi_991/1 -> cfblk6/1
  cfblk7/1 -> cyemi_991/1
  cyemi_992/1 -> cfblk7/1
  cfblk1/1 -> cyemi_992/1
  cyemi_993/1 -> cfblk8/1
  cfblk4/1 -> cyemi_993/1
  cyemi_994/1 -> cfblk9/1(cfblk1)
  cfblk13/1 -> cyemi_994/1
  cyemi_995/1 -> cfblk9/2(cfblk15)
  cfblk14/1 -> cyemi_995/1

== system sampleModel7288_pp_1_1/cfblk297 ==
  cfblk1 : Inport
  cfblk10 : Inport  Port=2
  cfblk11 : Inport  Port=3
  Action Port : ActionPort  ActionType=else
  cfblk13 : Delay
  cfblk14 : Delay
  cfblk3 : simulink/Discrete/Tapped Delay  vinit=0.0  samptime=-1  NumDelays=1  DelayOrder=Oldest  includeCurrent=off
  cfblk4 : Delay  ShowEnablePort=on
      settings: InputPortMap=u0,e6
  cfblk5 : simulink/Discrete/Transfer Fcn First Order  PoleZ=0.95  ICPrevOutput=0.0  DoSatur=off
      settings: SourceProductName=Simulink
  cfblk6 : Delay  ShowEnablePort=on
      settings: InputPortMap=u0,e6
  cfblk7 : Delay  ShowEnablePort=on
      settings: InputPortMap=u0,e6
  cfblk8 : simulink/Discrete/Transfer Fcn First Order  PoleZ=0.95  ICPrevOutput=0.0  DoSatur=off
      settings: SourceProductName=Simulink
  cfblk9 : simulink/Continuous/PID Controller (2DOF)  Controller=PID  TimeDomain=Discrete-time  SampleTime=-1  IntegratorMethod=Forward Euler  FilterMethod=Forward Euler  Form=Parallel  UseFilter=on  ControllerParametersSource=internal  P=1  I=1  D=0  N=100  b=1  c=1  InitialConditionSource=internal  InitialConditionForIntegrator=0  InitialConditionForFilter=0  ExternalReset=none  LimitOutput=off  UpperSaturationLimit=inf  LowerSaturationLimit=-inf  LinearizeAsGain=off  AntiWindupMode=none  Kb=1  TrackingMode=off  Kt=1  PParamMin=[]  PParamMax=[]  IParamMin=[]  IParamMax=[]  DParamMin=[]  DParamMax=[]  NParamMin=[]  NParamMax=[]  bParamMin=[]  bParamMax=[]  cParamMin=[]  cParamMax=[]  KbParamMin=[]  KbParamMax=[]  KtParamMin=[]  KtParamMax=[]  POutMin=[]  POutMax=[]  IOutMin=[]  IOutMax=[]  DOutMin=[]  DOutMax=[]  NOutMin=[]  NOutMax=[]  bOutMin=[]  bOutMax=[]  cOutMin=[]  cOutMax=[]  KbOutMin=[]  KbOutMax=[]  KtOutMin=[]  KtOutMax=[]  IntegratorOutMin=[]  IntegratorOutMax=[]  FilterOutMin=[]  FilterOutMax=[]  SumOutMin=[]  SumOutMax=[]  Sum1OutMin=[]  Sum1OutMax=[]  Sum2OutMin=[]  Sum2OutMax=[]  Sum3OutMin=[]  Sum3OutMax=[]  SumI1OutMin=[]  SumI1OutMax=[]  SumI2OutMin=[]  SumI2OutMax=[]  SumI3OutMin=[]  SumI3OutMax=[]  SumDOutMin=[]  SumDOutMax=[]  SaturationOutMin=[]  SaturationOutMax=[]  IntegratorContinuousStateAttributes=''  IntegratorStateMustResolveToSignalObject=off  IntegratorRTWStateStorageClass=Auto  FilterContinuousStateAttributes=''  FilterStateMustResolveToSignalObject=off  FilterRTWStateStorageClass=Auto  DifferentiatorICPrevScaledInput=0  DifferentiatorOutMin=[]  DifferentiatorOutMax=[]  FilterDiffOutCoefMin=[]  FilterDiffOutCoefMax=[]  SumDenOutMin=[]  SumDenOutMax=[]  SumNumOutMin=[]  SumNumOutMax=[]  ReciprocalOutMin=[]  ReciprocalOutMax=[]  DivideOutMin=[]  DivideOutMax=[]  TunerSelectOption=Transfer Function Based (PID Tuner App)
  cyemi_{1017..1029} (13 alike) : DataTypeConversion  OutDataTypeStr=double
  cfblk2 : Outport
  cfblk12 : Outport  Port=2
  wires:
  cfblk9/1 -> cyemi_1017/1, cyemi_1021/1
  cfblk3/1 -> cfblk2/1
  cfblk8/1 -> cyemi_1023/1, cyemi_1026/1
  cfblk7/1 -> cfblk12/1, cyemi_1024/1
  cyemi_1017/1 -> cfblk13/1
  cyemi_1018/1 -> cfblk14/1
  cfblk5/1 -> cyemi_1018/1
  cyemi_1019/1 -> cfblk3/1
  cfblk10/1 -> cyemi_1019/1
  cyemi_1020/1 -> cfblk4/1
  cfblk11/1 -> cyemi_1020/1
  cyemi_1021/1 -> cfblk4/2
  cyemi_1022/1 -> cfblk5/1
  cfblk4/1 -> cyemi_1022/1
  cyemi_1023/1 -> cfblk6/1
  cyemi_1024/1 -> cfblk6/2
  cyemi_1025/1 -> cfblk7/1
  cfblk13/1 -> cyemi_1025/1
  cyemi_1026/1 -> cfblk7/2
  cyemi_1027/1 -> cfblk8/1
  cfblk1/1 -> cyemi_1027/1
  cyemi_1028/1 -> cfblk9/1
  cfblk6/1 -> cyemi_1028/1
  cyemi_1029/1 -> cfblk9/2
  cfblk14/1 -> cyemi_1029/1

== system sampleModel7288_pp_1_1/cfblk298 ==
  cfblk1 : Inport
  cfblk10 : Inport  Port=2
  cfblk11 : Inport  Port=3
  cfblk12 : Inport  Port=4
  Action Port : ActionPort  ActionType=then
  cfblk16 : Delay
  cfblk3 : DiscreteFilter
  cfblk4 : Delay
  cfblk5 : DiscreteFir
  cfblk6 : simulink/Discrete/Tapped Delay  vinit=0.0  samptime=-1  NumDelays=1  DelayOrder=Oldest  includeCurrent=off
  cfblk7 : simulink/Discrete/Difference  ICPrevInput=0.0  OutMin=[]  OutMax=[]  OutDataTypeStr=double  OutputDataTypeScalingMode=double  OutDataType=fixdt(1, 16)  OutScaling=2^-10  DoSatur=off
  cfblk8 : simulink/Discrete/Transfer Fcn Real Zero  ZeroZ=0.75  ICPrevInput=0.0  DoSatur=off
      settings: SourceProductName=Simulink  SourceProductBaseCode=SL
  cfblk9 : simulink/Discrete/Difference  ICPrevInput=0.0  OutMin=[]  OutMax=[]  OutDataTypeStr=double  OutputDataTypeScalingMode=double  OutDataType=fixdt(1, 16)  OutScaling=2^-10  DoSatur=off
  cyemi_{1034..1041} (8 alike) : DataTypeConversion  OutDataTypeStr=double
  cfblk2 : Outport
  cfblk13 : Outport  Port=2
  cfblk14 : Outport  Port=3
  cfblk15 : Outport  Port=4
  wires:
  cfblk12/1 -> cfblk14/1
  cfblk9/1 -> cfblk15/1
  cfblk1/1 -> cfblk2/1
  cfblk3/1 -> cfblk13/1
  cyemi_1034/1 -> cfblk16/1
  cfblk5/1 -> cyemi_1034/1
  cyemi_1035/1 -> cfblk3/1
  cfblk7/1 -> cyemi_1035/1
  cyemi_1036/1 -> cfblk4/1
  cfblk16/1 -> cyemi_1036/1
  cyemi_1037/1 -> cfblk5/1
  cfblk6/1 -> cyemi_1037/1
  cyemi_1038/1 -> cfblk6/1
  cfblk4/1 -> cyemi_1038/1
  cyemi_1039/1 -> cfblk7/1
  cfblk8/1 -> cyemi_1039/1
  cyemi_1040/1 -> cfblk8/1
  cfblk10/1 -> cyemi_1040/1
  cyemi_1041/1 -> cfblk9/1
  cfblk11/1 -> cyemi_1041/1

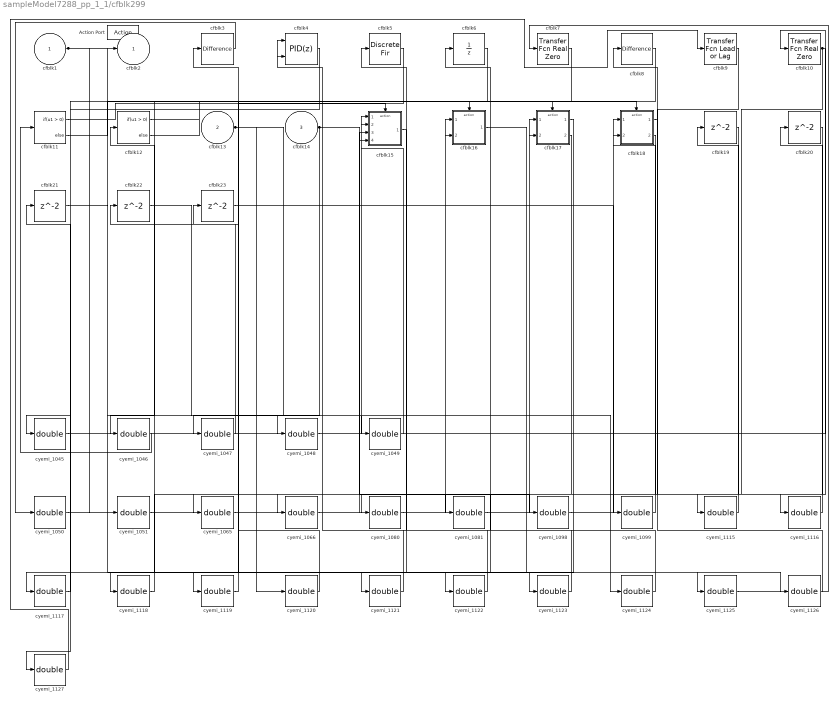
== system sampleModel7288_pp_1_1/cfblk299 ==
  cfblk1 : Inport
  cfblk13 : Inport  Port=2
  cfblk14 : Inport  Port=3
  Action Port : ActionPort  ActionType=else
  cfblk10 : simulink/Discrete/Transfer Fcn Real Zero  ZeroZ=0.75  ICPrevInput=0.0  DoSatur=off
      settings: SourceProductName=Simulink  SourceProductBaseCode=SL
  cfblk11 : If  SampleTime=1
  cfblk12 : If  SampleTime=1
  cfblk15 : Subsystem  TreatAsAtomicUnit=on
  cfblk16 : Subsystem  TreatAsAtomicUnit=on
  cfblk17 : Subsystem  TreatAsAtomicUnit=on
  cfblk18 : Subsystem  TreatAsAtomicUnit=on
  cfblk{19..23} (5 alike) : Delay
  cfblk3 : simulink/Discrete/Difference  ICPrevInput=0.0  OutMin=[]  OutMax=[]  OutDataTypeStr=double  OutputDataTypeScalingMode=double  OutDataType=fixdt(1, 16)  OutScaling=2^-10  DoSatur=off
  cfblk4 : simulink/Continuous/PID Controller (2DOF)  Controller=PID  TimeDomain=Discrete-time  SampleTime=-1  IntegratorMethod=Forward Euler  FilterMethod=Forward Euler  Form=Parallel  UseFilter=on  ControllerParametersSource=internal  P=1  I=1  D=0  N=100  b=1  c=1  InitialConditionSource=internal  InitialConditionForIntegrator=0  InitialConditionForFilter=0  ExternalReset=none  LimitOutput=off  UpperSaturationLimit=inf  LowerSaturationLimit=-inf  LinearizeAsGain=off  AntiWindupMode=none  Kb=1  TrackingMode=off  Kt=1  PParamMin=[]  PParamMax=[]  IParamMin=[]  IParamMax=[]  DParamMin=[]  DParamMax=[]  NParamMin=[]  NParamMax=[]  bParamMin=[]  bParamMax=[]  cParamMin=[]  cParamMax=[]  KbParamMin=[]  KbParamMax=[]  KtParamMin=[]  KtParamMax=[]  POutMin=[]  POutMax=[]  IOutMin=[]  IOutMax=[]  DOutMin=[]  DOutMax=[]  NOutMin=[]  NOutMax=[]  bOutMin=[]  bOutMax=[]  cOutMin=[]  cOutMax=[]  KbOutMin=[]  KbOutMax=[]  KtOutMin=[]  KtOutMax=[]  IntegratorOutMin=[]  IntegratorOutMax=[]  FilterOutMin=[]  FilterOutMax=[]  SumOutMin=[]  SumOutMax=[]  Sum1OutMin=[]  Sum1OutMax=[]  Sum2OutMin=[]  Sum2OutMax=[]  Sum3OutMin=[]  Sum3OutMax=[]  SumI1OutMin=[]  SumI1OutMax=[]  SumI2OutMin=[]  SumI2OutMax=[]  SumI3OutMin=[]  SumI3OutMax=[]  SumDOutMin=[]  SumDOutMax=[]  SaturationOutMin=[]  SaturationOutMax=[]  IntegratorContinuousStateAttributes=''  IntegratorStateMustResolveToSignalObject=off  IntegratorRTWStateStorageClass=Auto  FilterContinuousStateAttributes=''  FilterStateMustResolveToSignalObject=off  FilterRTWStateStorageClass=Auto  DifferentiatorICPrevScaledInput=0  DifferentiatorOutMin=[]  DifferentiatorOutMax=[]  FilterDiffOutCoefMin=[]  FilterDiffOutCoefMax=[]  SumDenOutMin=[]  SumDenOutMax=[]  SumNumOutMin=[]  SumNumOutMax=[]  ReciprocalOutMin=[]  ReciprocalOutMax=[]  DivideOutMin=[]  DivideOutMax=[]  TunerSelectOption=Transfer Function Based (PID Tuner App)
  cfblk5 : DiscreteFir
  cfblk6 : UnitDelay  SampleTime=-1
  cfblk7 : simulink/Discrete/Transfer Fcn Real Zero  ZeroZ=0.75  ICPrevInput=0.0  DoSatur=off
      settings: SourceProductName=Simulink  SourceProductBaseCode=SL
  cfblk8 : simulink/Discrete/Difference  ICPrevInput=0.0  OutMin=[]  OutMax=[]  OutDataTypeStr=double  OutputDataTypeScalingMode=double  OutDataType=fixdt(1, 16)  OutScaling=2^-10  DoSatur=off
  cfblk9 : simulink/Discrete/Transfer Fcn Lead or Lag  PoleZ=0.95  ZeroZ=0.75  ICPrevOutput=0.0  ICPrevInput=0.0  DoSatur=off
      settings: SourceProductName=Simulink  SourceProductBaseCode=SL
  cyemi_{1045..1051,1065..1066,1080..1081,1098..1099,1115..1127} (26 alike) : DataTypeConversion  OutDataTypeStr=double
  cfblk2 : Outport
  wires:
  cfblk14/1 -> cyemi_1065/1, cyemi_1098/1
  cfblk13/1 -> cyemi_1120/1, cyemi_1124/1
  cfblk10/1 -> cyemi_1115/1, cyemi_1116/1
  cfblk1/1 -> cfblk2/1, cyemi_1051/1, cyemi_1126/1
  cfblk11/1 -> cfblk15/Action
  cfblk11/2 -> cfblk16/Action
  cfblk12/1 -> cfblk17/Action
  cfblk12/2 -> cfblk18/Action
  cyemi_1045/1 -> cfblk10/1
  cfblk4/1 -> cyemi_1045/1
  cyemi_1046/1 -> cfblk11/1
  cfblk6/1 -> cyemi_1046/1
  cyemi_1047/1 -> cfblk12/1
  cfblk8/1 -> cyemi_1047/1
  cyemi_1048/1 -> cfblk15/1(cfblk1)
  cfblk21/1 -> cyemi_1048/1
  cyemi_1049/1 -> cfblk15/2(cfblk13)
  cfblk22/1 -> cyemi_1049/1
  cyemi_1050/1 -> cfblk15/3(cfblk14)
  cfblk3/1 -> cyemi_1050/1
  cyemi_1051/1 -> cfblk15/4(cfblk15)
  cyemi_1065/1 -> cfblk16/1(cfblk1)
  cyemi_1066/1 -> cfblk16/2(cfblk15)
  cfblk20/1 -> cyemi_1066/1
  cyemi_1080/1 -> cfblk17/1(cfblk1)
  cfblk9/1 -> cyemi_1080/1
  cyemi_1081/1 -> cfblk17/2(cfblk16)
  cfblk18/1(cfblk2) -> cyemi_1081/1
  cyemi_1098/1 -> cfblk18/1(cfblk1)
  cyemi_1099/1 -> cfblk18/2(cfblk15)
  cfblk23/1 -> cyemi_1099/1
  cyemi_1115/1 -> cfblk19/1
  cyemi_1116/1 -> cfblk20/1
  cyemi_1117/1 -> cfblk21/1
  cfblk17/1(cfblk2) -> cyemi_1117/1
  cyemi_1118/1 -> cfblk22/1
  cfblk17/2(cfblk17) -> cyemi_1118/1
  cyemi_1119/1 -> cfblk23/1
  cfblk5/1 -> cyemi_1119/1
  cyemi_1120/1 -> cfblk3/1
  cyemi_1121/1 -> cfblk4/1
  cfblk15/1(cfblk2) -> cyemi_1121/1
  cyemi_1122/1 -> cfblk4/2
  cfblk19/1 -> cyemi_1122/1
  cyemi_1123/1 -> cfblk5/1
  cfblk18/2(cfblk16) -> cyemi_1123/1
  cyemi_1124/1 -> cfblk6/1
  cyemi_1125/1 -> cfblk7/1
  cfblk16/1(cfblk2) -> cyemi_1125/1
  cyemi_1126/1 -> cfblk8/1
  cyemi_1127/1 -> cfblk9/1
  cfblk7/1 -> cyemi_1127/1

== system sampleModel7288_pp_1_1/cfblk300 ==
  cfblk1 : Inport
  Action Port : ActionPort  ActionType=then
  cfblk3 : DiscreteFilter
  cfblk4 : Subsystem  TreatAsAtomicUnit=on
  cfblk5 : simulink/Discrete/Transfer Fcn First Order  PoleZ=0.95  ICPrevOutput=0.0  DoSatur=off
      settings: SourceProductName=Simulink
  cfblk6 : simulink/Discrete/Tapped Delay  vinit=0.0  samptime=-1  NumDelays=1  DelayOrder=Oldest  includeCurrent=off
  cfblk7 : simulink/Discrete/Tapped Delay  vinit=0.0  samptime=-1  NumDelays=1  DelayOrder=Oldest  includeCurrent=off
  cfblk8 : simulink/Discrete/Difference  ICPrevInput=0.0  OutMin=[]  OutMax=[]  OutDataTypeStr=double  OutputDataTypeScalingMode=double  OutDataType=fixdt(1, 16)  OutScaling=2^-10  DoSatur=off
  cfblk9 : Delay
  cyemi_{1132..1138} (7 alike) : DataTypeConversion  OutDataTypeStr=double
  emi_3 : Subsystem  TreatAsAtomicUnit=on
  cfblk2 : Outport
  wires:
  cfblk3/1 -> cfblk2/1
  cyemi_1132/1 -> cfblk3/1
  cfblk1/1 -> cyemi_1132/1
  cfblk9/1 -> cyemi_1133/1
  cyemi_1134/1 -> cfblk5/1
  cfblk8/1 -> cyemi_1134/1
  cyemi_1135/1 -> cfblk6/1
  cyemi_1136/1 -> cfblk7/1
  cfblk6/1 -> cyemi_1136/1
  cyemi_1137/1 -> cfblk8/1
  cfblk7/1 -> cyemi_1137/1
  cyemi_1138/1 -> cfblk9/1
  cfblk5/1 -> cyemi_1138/1
  cyemi_1133/1 -> cfblk4/1(emi_1)
  cfblk4/1(emi_2) -> cyemi_1135/1

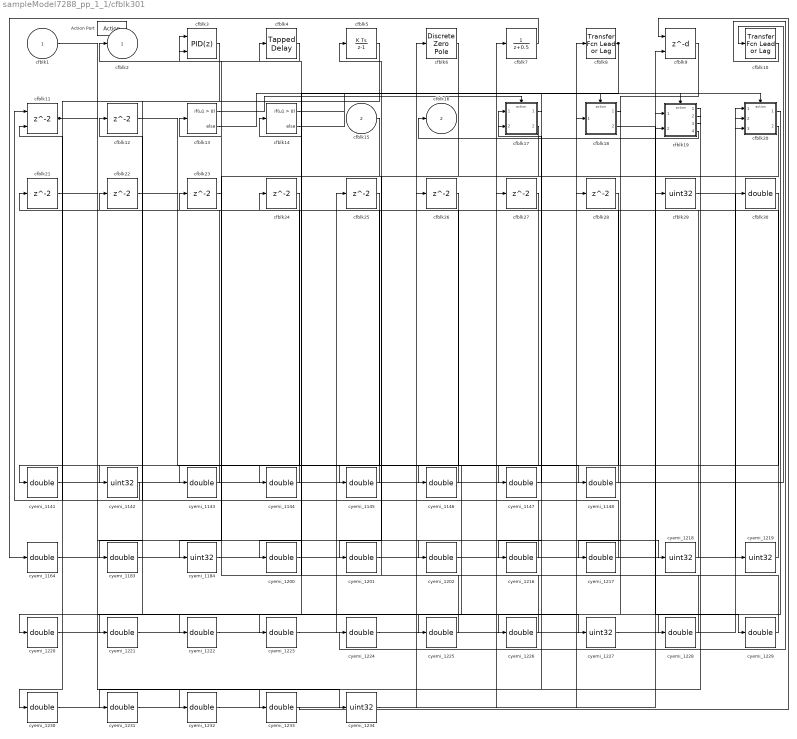
== system sampleModel7288_pp_1_1/cfblk301 ==
  cfblk1 : Inport
  cfblk15 : Inport  Port=2
  Action Port : ActionPort  ActionType=else
  cfblk10 : simulink/Discrete/Transfer Fcn Lead or Lag  PoleZ=0.95  ZeroZ=0.75  ICPrevOutput=0.0  ICPrevInput=0.0  DoSatur=off
      settings: SourceProductName=Simulink  SourceProductBaseCode=SL
  cfblk11 : Delay  ShowEnablePort=on
      settings: InputPortMap=u0,e6
  cfblk{12,21..28} (9 alike) : Delay
  cfblk13 : If  SampleTime=1
  cfblk14 : If  SampleTime=1
  cfblk17 : Subsystem  TreatAsAtomicUnit=on
  cfblk18 : Subsystem  TreatAsAtomicUnit=on
  cfblk19 : Subsystem  TreatAsAtomicUnit=on
  cfblk20 : Subsystem  TreatAsAtomicUnit=on
  cfblk29 : DataTypeConversion  OutDataTypeStr=uint32
  cfblk3 : simulink/Continuous/PID Controller (2DOF)  Controller=PID  TimeDomain=Discrete-time  SampleTime=-1  IntegratorMethod=Forward Euler  FilterMethod=Forward Euler  Form=Parallel  UseFilter=on  ControllerParametersSource=internal  P=1  I=1  D=0  N=100  b=1  c=1  InitialConditionSource=internal  InitialConditionForIntegrator=0  InitialConditionForFilter=0  ExternalReset=none  LimitOutput=off  UpperSaturationLimit=inf  LowerSaturationLimit=-inf  LinearizeAsGain=off  AntiWindupMode=none  Kb=1  TrackingMode=off  Kt=1  PParamMin=[]  PParamMax=[]  IParamMin=[]  IParamMax=[]  DParamMin=[]  DParamMax=[]  NParamMin=[]  NParamMax=[]  bParamMin=[]  bParamMax=[]  cParamMin=[]  cParamMax=[]  KbParamMin=[]  KbParamMax=[]  KtParamMin=[]  KtParamMax=[]  POutMin=[]  POutMax=[]  IOutMin=[]  IOutMax=[]  DOutMin=[]  DOutMax=[]  NOutMin=[]  NOutMax=[]  bOutMin=[]  bOutMax=[]  cOutMin=[]  cOutMax=[]  KbOutMin=[]  KbOutMax=[]  KtOutMin=[]  KtOutMax=[]  IntegratorOutMin=[]  IntegratorOutMax=[]  FilterOutMin=[]  FilterOutMax=[]  SumOutMin=[]  SumOutMax=[]  Sum1OutMin=[]  Sum1OutMax=[]  Sum2OutMin=[]  Sum2OutMax=[]  Sum3OutMin=[]  Sum3OutMax=[]  SumI1OutMin=[]  SumI1OutMax=[]  SumI2OutMin=[]  SumI2OutMax=[]  SumI3OutMin=[]  SumI3OutMax=[]  SumDOutMin=[]  SumDOutMax=[]  SaturationOutMin=[]  SaturationOutMax=[]  IntegratorContinuousStateAttributes=''  IntegratorStateMustResolveToSignalObject=off  IntegratorRTWStateStorageClass=Auto  FilterContinuousStateAttributes=''  FilterStateMustResolveToSignalObject=off  FilterRTWStateStorageClass=Auto  DifferentiatorICPrevScaledInput=0  DifferentiatorOutMin=[]  DifferentiatorOutMax=[]  FilterDiffOutCoefMin=[]  FilterDiffOutCoefMax=[]  SumDenOutMin=[]  SumDenOutMax=[]  SumNumOutMin=[]  SumNumOutMax=[]  ReciprocalOutMin=[]  ReciprocalOutMax=[]  DivideOutMin=[]  DivideOutMax=[]  TunerSelectOption=Transfer Function Based (PID Tuner App)
  cfblk30 : DataTypeConversion  OutDataTypeStr=double
  cfblk4 : simulink/Discrete/Tapped Delay  vinit=0.0  samptime=-1  NumDelays=1  DelayOrder=Oldest  includeCurrent=off
  cfblk5 : DiscreteIntegrator  SampleTime=-1  OutDataTypeStr=double  ICPrevOutput=DiscIntNeverNeededParam  ICPrevScaledInput=DiscIntNeverNeededParam
  cfblk6 : DiscreteZeroPole  Poles=[0 0.5]  Gain=1  SampleTime=-1
  cfblk7 : DiscreteTransferFcn
  cfblk8 : simulink/Discrete/Transfer Fcn Lead or Lag  PoleZ=0.95  ZeroZ=0.75  ICPrevOutput=0.0  ICPrevInput=0.0  DoSatur=off
      settings: SourceProductName=Simulink  SourceProductBaseCode=SL
  cfblk9 : Delay  DelayLengthSource=Input port
      settings: InputPortMap=u0,p1
  cyemi_{1141,1143..1148,1164,1183,1200..1202,1216..1217,1220..1226,1228..1233} (27 alike) : DataTypeConversion  OutDataTypeStr=double
  cyemi_{1142,1184,1218..1219,1227,1234} (6 alike) : DataTypeConversion  OutDataTypeStr=uint32
  cfblk2 : Outport
  cfblk16 : Outport  Port=2
  wires:
  cfblk4/1 -> cfblk2/1
  cfblk11/1 -> cyemi_1218/1, cyemi_1227/1, cyemi_1234/1
  cfblk19/4(cfblk14) -> cfblk16/1
  cfblk8/1 -> cyemi_1144/1, cyemi_1216/1
  cfblk13/1 -> cfblk17/Action
  cfblk13/2 -> cfblk18/Action
  cfblk14/1 -> cfblk19/Action
  cfblk14/2 -> cfblk20/Action
  cyemi_1141/1 -> cfblk10/1
  cfblk30/1 -> cyemi_1141/1
  cyemi_1142/1 -> cfblk11/1
  cfblk24/1 -> cyemi_1142/1
  cyemi_1143/1 -> cfblk11/2
  cfblk17/2(cfblk17) -> cyemi_1143/1
  cyemi_1144/1 -> cfblk12/1
  cyemi_1145/1 -> cfblk13/1
  cfblk25/1 -> cyemi_1145/1
  cyemi_1146/1 -> cfblk14/1
  cfblk27/1 -> cyemi_1146/1
  cyemi_1147/1 -> cfblk17/1(cfblk1)
  cfblk22/1 -> cyemi_1147/1
  cyemi_1148/1 -> cfblk17/2(cfblk16)
  cfblk12/1 -> cyemi_1148/1
  cyemi_1164/1 -> cfblk18/1(cfblk1)
  cfblk7/1 -> cyemi_1164/1
  cyemi_1183/1 -> cfblk19/1(cfblk1)
  cfblk26/1 -> cyemi_1183/1
  cyemi_1184/1 -> cfblk19/2(cfblk11)
  cfblk23/1 -> cyemi_1184/1
  cyemi_1200/1 -> cfblk20/1(cfblk1)
  cfblk15/1 -> cyemi_1200/1
  cyemi_1201/1 -> cfblk20/2(cfblk12)
  cfblk6/1 -> cyemi_1201/1
  cyemi_1202/1 -> cfblk20/3(cfblk13)
  cfblk21/1 -> cyemi_1202/1
  cyemi_1216/1 -> cfblk21/1
  cyemi_1217/1 -> cfblk22/1
  cfblk9/1 -> cyemi_1217/1
  cyemi_1218/1 -> cfblk23/1
  cyemi_1219/1 -> cfblk24/1
  cfblk29/1 -> cyemi_1219/1
  cyemi_1220/1 -> cfblk25/1
  cfblk18/1(cfblk2) -> cyemi_1220/1
  cyemi_1221/1 -> cfblk26/1
  cfblk5/1 -> cyemi_1221/1
  cyemi_1222/1 -> cfblk27/1
  cfblk20/1(cfblk2) -> cyemi_1222/1
  cyemi_1223/1 -> cfblk28/1
  cfblk20/2(cfblk14) -> cyemi_1223/1
  cyemi_1224/1 -> cfblk29/1
  cfblk10/1 -> cyemi_1224/1
  cyemi_1225/1 -> cfblk3/1
  cfblk28/1 -> cyemi_1225/1
  cyemi_1226/1 -> cfblk3/2
  cfblk1/1 -> cyemi_1226/1
  cyemi_1227/1 -> cfblk30/1
  cyemi_1228/1 -> cfblk4/1
  cfblk19/1(cfblk2) -> cyemi_1228/1
  cyemi_1229/1 -> cfblk5/1
  cfblk18/2(cfblk15) -> cyemi_1229/1
  cyemi_1230/1 -> cfblk6/1
  cfblk3/1 -> cyemi_1230/1
  cyemi_1231/1 -> cfblk7/1
  cfblk19/3(cfblk13) -> cyemi_1231/1
  cyemi_1232/1 -> cfblk8/1
  cfblk19/2(cfblk12) -> cyemi_1232/1
  cyemi_1233/1 -> cfblk9/1
  cfblk17/1(cfblk2) -> cyemi_1233/1
  cyemi_1234/1 -> cfblk9/2
